simulink model "spwm"  (R2024a)
settings: Solver=FixedStepAuto  StartTime=0.0  StopTime=0.1  FixedStep=1e-5  RelTol=1e-3
libraries: simulink x7
settings Model: Creator=ammarabdulrasheed  LastModifiedBy=ammarabdulrasheed

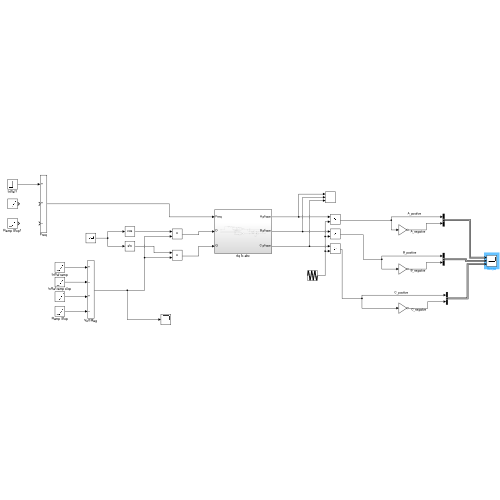
[thumbnail: Simulink's stored preview of the top-level diagram]
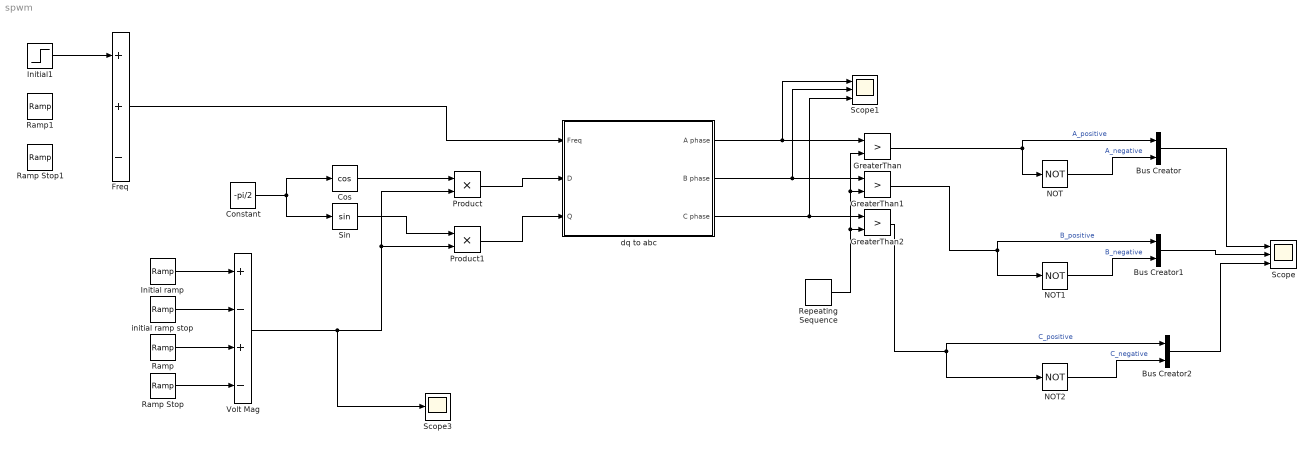
== system spwm ==
  Bus Creator : BusCreator  Inputs=2
  Bus Creator1 : BusCreator  Inputs=2
  Bus Creator2 : BusCreator  Inputs=2
  Constant : Constant  Value=-pi/2
  Cos : Trigonometry  Operator=cos
  Freq : Sum  Inputs=++-
  GreaterThan : RelationalOperator  Operator=>  OutDataTypeStr=boolean  RndMeth=Simplest  InputSameDT=off
  GreaterThan1 : RelationalOperator  Operator=>  OutDataTypeStr=boolean  RndMeth=Simplest  InputSameDT=off
  GreaterThan2 : RelationalOperator  Operator=>  OutDataTypeStr=boolean  RndMeth=Simplest  InputSameDT=off
  Initial ramp : simulink/Sources/Ramp  slope=100000  start=0  InitialOutput=0
  Initial1 : Step  Time=0  After=50  SampleTime=0
  NOT : Logic  Operator=NOT  IconShape=distinctive  AllPortsSameDT=off  OutDataTypeStr=boolean
  NOT1 : Logic  Operator=NOT  IconShape=distinctive  AllPortsSameDT=off  OutDataTypeStr=boolean
  NOT2 : Logic  Operator=NOT  IconShape=distinctive  AllPortsSameDT=off  OutDataTypeStr=boolean
  Product : Product
  Product1 : Product
  Ramp : simulink/Sources/Ramp  slope=4/0.1  start=0  InitialOutput=0
  Ramp Stop : simulink/Sources/Ramp  slope=40  start=0.1  InitialOutput=0
  Ramp Stop1 : simulink/Sources/Ramp  slope=25  start=3  InitialOutput=0
  Ramp1 : simulink/Sources/Ramp  slope=25  start=1  InitialOutput=0
  Repeating Sequence : simulink/Sources/Repeating Sequence  rep_seq_t=[0 1 2 3 4]*1e-4  rep_seq_y=[0 1 0 -1 0]
  Scope : Scope  NumInputPorts=3
  Scope1 : Scope  NumInputPorts=3
  Scope3 : Scope
  Sin : Trigonometry
  Volt Mag : Sum  Inputs=+-+-
  dq to abc : Subsystem
  initial ramp stop : simulink/Sources/Ramp  slope=100000  start=1e-5  InitialOutput=0
  wires:
  Product/1 -> dq to abc/2(D)
  Sin/1 -> Product1/1
  Freq/1 -> dq to abc/1(Freq)
  Initial1/1 -> Freq/1
  Constant/1 -> Sin/1, Cos/1
  Product1/1 -> dq to abc/3(Q)
  Initial ramp/1 -> Volt Mag/1
  Volt Mag/1 -> Scope3/1, Product1/2, Product/2
  initial ramp stop/1 -> Volt Mag/2
  Cos/1 -> Product/1
  dq to abc/1(A phase) -> Scope1/1, GreaterThan/1
  dq to abc/2(B phase) -> Scope1/2, GreaterThan1/1
  dq to abc/3(C phase) -> Scope1/3, GreaterThan2/1
  Repeating Sequence/1 -> GreaterThan/2, GreaterThan1/2, GreaterThan2/2
  GreaterThan/1 -> Bus Creator/1, NOT/1  "A_positive"
  NOT/1 -> Bus Creator/2  "A_negative"
  GreaterThan1/1 -> Bus Creator1/1, NOT1/1  "B_positive"
  NOT1/1 -> Bus Creator1/2  "B_negative"
  GreaterThan2/1 -> Bus Creator2/1, NOT2/1  "C_positive"
  NOT2/1 -> Bus Creator2/2  "C_negative"
  Bus Creator/1 -> Scope/1
  Bus Creator1/1 -> Scope/2
  Bus Creator2/1 -> Scope/3
  Ramp/1 -> Volt Mag/3
  Ramp Stop/1 -> Volt Mag/4

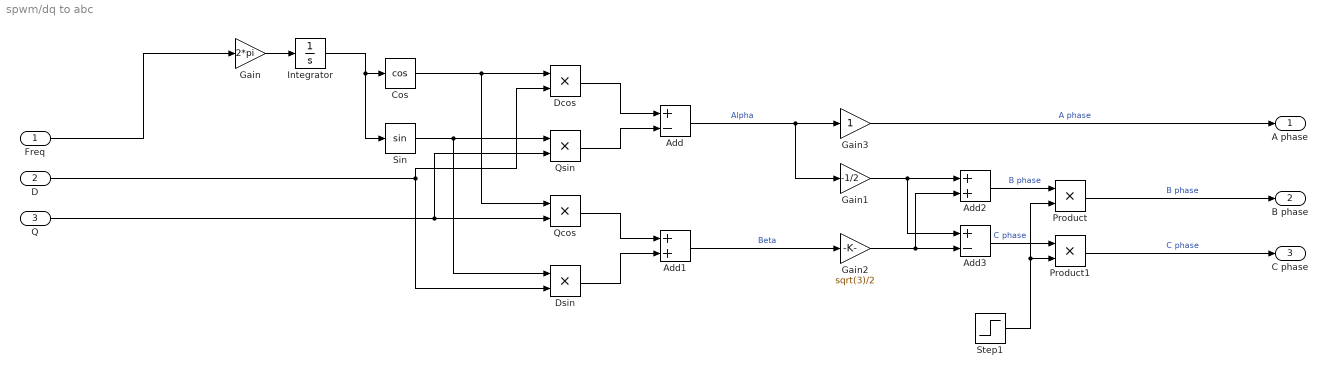
== system spwm/dq to abc ==
  Freq : Inport
  D : Inport  Port=2
  Q : Inport  Port=3
  Add : Sum  Inputs=+-
  Add1 : Sum
  Add2 : Sum
  Add3 : Sum  Inputs=+-
  Cos : Trigonometry  Operator=cos
  Dcos : Product
  Dsin : Product
  Gain : Gain  Gain=2*pi
  Gain1 : Gain  Gain=-1/2
  Gain2 : Gain  Gain=sqrt(3)/2
  Gain3 : Gain
  Integrator : Integrator
  Product : Product
  Product1 : Product
  Qcos : Product
  Qsin : Product
  Sin : Trigonometry
  Step1 : Step  Time=0  SampleTime=0
  A phase : Outport
  B phase : Outport  Port=2
  C phase : Outport  Port=3
  wires:
  Product/1 -> B phase/1  "B phase"
  Add1/1 -> Gain2/1  "Beta"
  Product1/1 -> C phase/1  "C phase"
  D/1 -> Dsin/2, Dcos/2
  Dsin/1 -> Add1/2
  Freq/1 -> Gain/1
  Step1/1 -> Product1/2, Product/2
  Q/1 -> Qcos/2, Qsin/2
  Dcos/1 -> Add/1
  Gain/1 -> Integrator/1
  Gain3/1 -> A phase/1  "A phase"
  Cos/1 -> Qcos/1, Dcos/1
  Add2/1 -> Product/1  "B phase"
  Gain2/1 -> Add3/2, Add2/2
  Integrator/1 -> Sin/1, Cos/1
  Add3/1 -> Product1/1  "C phase"
  Sin/1 -> Dsin/1, Qsin/1
  Gain1/1 -> Add3/1, Add2/1
  Qsin/1 -> Add/2
  Qcos/1 -> Add1/1
  Add/1 -> Gain1/1, Gain3/1  "Alpha"
